simulink model "Passive_balancing"  (R2021a)
settings: Solver=ode23t  StartTime=0.0  StopTime=inf  FixedStep=0.01  MaxStep=0.01  RelTol=1e-3
undefined symbols (not defined in the file): Ion, Lithium
libraries: spsBatteryLib x3, spsIGBTLib x3, spsSeriesRLCBranchLib x3, spspowerguiLib x2
settings Model: PacingRate=79  Creator=AHMED  LastModifiedBy=AHMED

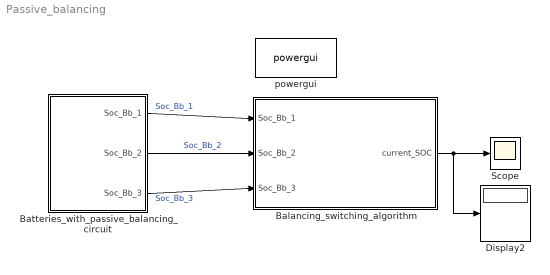
== system Passive_balancing ==
  Balancing_switching_algorithm : Subsystem
  Batteries_with_passive_balancing_circuit : Subsystem  mask{Battery_1_Soc=25, Battery_2_Soc=30, Battery_3_Soc=35}
  Display2 : Display
  Scope : Scope
  powergui : spspowerguiLib/powergui  Priority=1  SimulationMode=Continuous  SampleTime=50e-6  frequency=60  Iterations=50  frequencyindice=0  Pbase=100e6  ErrMax=1e-4  UnitsV=kV  UnitsW=MW  buscounter=0  FunctionMessages=off  echomessages=off  EnableUseOfTLC=off  CurrentSourceSwitches=off  DisableSnubberDevices=off  DisableRonSwitches=off  DisableVfSwitches=off  DisplayEquations=off  AutomaticDiscreteSolvers=off  SolverType=Tustin/Backward Euler (TBE)  Interpol=off  ExternalGateDelay=off  methode=off  Ts=100  x0status=blocks  SPID=on  SwTol=0  HookPort=off  NonlinearTolerance=1e-4  nMaxIteration=100  ContinueOnMaxIteration=off  RestoreLinks=warning  ResistiveCurrentMeasurement=off  Frange=[0:2:500]  Ylog=off  Xlog=on  ShowGrid=off  save=off  variable=ZData  structure=0  ZoomFFT=off  StartTime=0.0  cycles=1  DisplayStyle=1  fundamental=60  FreqAxis=off  MaxFrequency=1000  frequencyindicesteady=1  RmsSteady=1  display=off
  wires:
  Balancing_switching_algorithm/1(current_SOC) -> Display2/1, Scope/1
  Batteries_with_passive_balancing_circuit/1(Soc_Bb_1) -> Balancing_switching_algorithm/1(Soc_Bb_1)  "Soc_Bb_1"
  Batteries_with_passive_balancing_circuit/2(Soc_Bb_2) -> Balancing_switching_algorithm/2(Soc_Bb_2)  "Soc_Bb_2"
  Batteries_with_passive_balancing_circuit/3(Soc_Bb_3) -> Balancing_switching_algorithm/3(Soc_Bb_3)  "Soc_Bb_3"

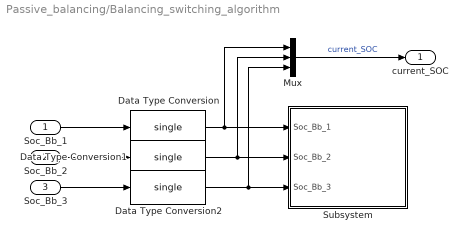
== system Passive_balancing/Balancing_switching_algorithm ==
  Soc_Bb_1 : Inport
  Soc_Bb_2 : Inport  Port=2
  Soc_Bb_3 : Inport  Port=3
  Data Type Conversion : DataTypeConversion  OutDataTypeStr=single
  Data Type Conversion1 : DataTypeConversion  OutDataTypeStr=single
  Data Type Conversion2 : DataTypeConversion  OutDataTypeStr=single
  Mux : Mux  Inputs=3
  Subsystem : Subsystem
  current_SOC : Outport
  wires:
  Data Type Conversion/1 -> Subsystem/1(Soc_Bb_1), Mux/1
  Data Type Conversion1/1 -> Subsystem/2(Soc_Bb_2), Mux/2
  Soc_Bb_3/1 -> Data Type Conversion2/1
  Data Type Conversion2/1 -> Subsystem/3(Soc_Bb_3), Mux/3
  Soc_Bb_2/1 -> Data Type Conversion1/1
  Mux/1 -> current_SOC/1  "current_SOC"
  Soc_Bb_1/1 -> Data Type Conversion/1

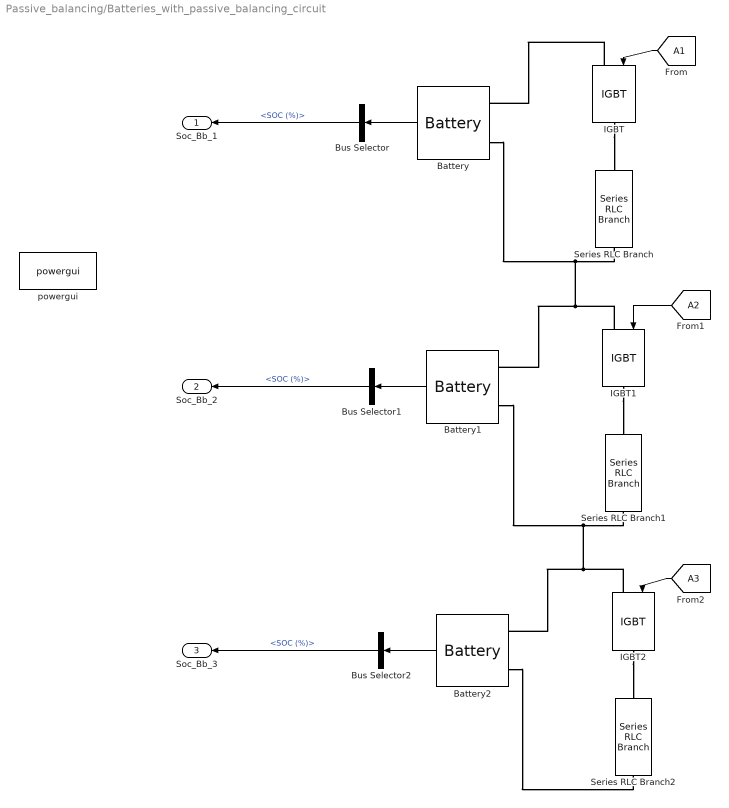
== system Passive_balancing/Batteries_with_passive_balancing_circuit ==
  Battery : spsBatteryLib/Battery  BatType=Lithium-Ion  ShowTempParam=off  ThermalPreset=no  ShowAgeParam=off  NomV=3.7  NomQ=5.4  SOC=Battery_1_Soc  Batt_Tr=30  PresetModel=on  MaxQ=5.4  MinV=2.775  FullV=4.3068  Dis_rate=2.3478  R=0.0068519  Normal_OP=4.8835  expZone="[3.9974      0.2653]"  current=[6.5 13 32.5]  Units=Time  Tci=20  NomT=20  T2=-30  MaxQ2=4.8  FullV2=7.1  Normal_OP2=5.655  expZone2="[6.58           1]"  Rca=0.6  ti=2000  Dp=0  Neq0=0  Tsim=1e6  Ta1=25  Qeol=5.4*0.9  Reol=0.013333*1.2  Char_age=[2.3478, 3]  Dis_age=[2.3478, 10]  N1=1500  N2=10500  N3=1000  N4=1400  Ta2=45  N5=950
  Battery1 : spsBatteryLib/Battery  BatType=Lithium-Ion  ShowTempParam=off  ThermalPreset=no  ShowAgeParam=off  NomV=3.7  NomQ=5.4  SOC=Battery_2_Soc  Batt_Tr=30  PresetModel=on  MaxQ=5.4  MinV=2.775  FullV=4.3068  Dis_rate=2.3478  R=0.0068519  Normal_OP=4.8835  expZone="[3.9974      0.2653]"  current=[6.5 13 32.5]  Units=Time  Tci=20  NomT=20  T2=-30  MaxQ2=4.8  FullV2=7.1  Normal_OP2=5.655  expZone2="[6.58           1]"  Rca=0.6  ti=2000  Dp=0  Neq0=0  Tsim=1e6  Ta1=25  Qeol=5.4*0.9  Reol=0.013333*1.2  Char_age=[2.3478, 3]  Dis_age=[2.3478, 10]  N1=1500  N2=10500  N3=1000  N4=1400  Ta2=45  N5=950
  Battery2 : spsBatteryLib/Battery  BatType=Lithium-Ion  ShowTempParam=off  ThermalPreset=no  ShowAgeParam=off  NomV=3.7  NomQ=5.4  SOC=Battery_3_Soc  Batt_Tr=30  PresetModel=on  MaxQ=5.4  MinV=2.775  FullV=4.3068  Dis_rate=2.3478  R=0.0068519  Normal_OP=4.8835  expZone="[3.9974      0.2653]"  current=[6.5 13 32.5]  Units=Time  Tci=20  NomT=20  T2=-30  MaxQ2=4.8  FullV2=7.1  Normal_OP2=5.655  expZone2="[6.58           1]"  Rca=0.6  ti=2000  Dp=0  Neq0=0  Tsim=1e6  Ta1=25  Qeol=5.4*0.9  Reol=0.013333*1.2  Char_age=[2.3478, 3]  Dis_age=[2.3478, 10]  N1=1500  N2=10500  N3=1000  N4=1400  Ta2=45  N5=950
  Bus Selector : BusSelector  OutputSignals=SOC (%)
  Bus Selector1 : BusSelector  OutputSignals=SOC (%)
  Bus Selector2 : BusSelector  OutputSignals=SOC (%)
  IGBT : spsIGBTLib/IGBT  Ron=0.001  Lon=0  Vf=1  Tf=1e-6  Tt=2e-6  IC=0  Rs=1e5  Cs=inf  Measurements=off
  IGBT1 : spsIGBTLib/IGBT  Ron=0.001  Lon=0  Vf=1  Tf=1e-6  Tt=2e-6  IC=0  Rs=1e5  Cs=inf  Measurements=off
  IGBT2 : spsIGBTLib/IGBT  Ron=0.001  Lon=0  Vf=1  Tf=1e-6  Tt=2e-6  IC=0  Rs=1e5  Cs=inf  Measurements=off
  Series RLC Branch : spsSeriesRLCBranchLib/Series RLC Branch  LConnTagsString=__new0  RConnTagsString=__new0  BranchType=R  Resistance=1  Inductance=1e-3  SetiL0=off  InitialCurrent=0  Capacitance=1e-6  Setx0=off  InitialVoltage=0  Measurements=None
  Series RLC Branch1 : spsSeriesRLCBranchLib/Series RLC Branch  LConnTagsString=__new0  RConnTagsString=__new0  BranchType=R  Resistance=1  Inductance=1e-3  SetiL0=off  InitialCurrent=0  Capacitance=1e-6  Setx0=off  InitialVoltage=0  Measurements=None
  Series RLC Branch2 : spsSeriesRLCBranchLib/Series RLC Branch  LConnTagsString=__new0  RConnTagsString=__new0  BranchType=R  Resistance=1  Inductance=1e-3  SetiL0=off  InitialCurrent=0  Capacitance=1e-6  Setx0=off  InitialVoltage=0  Measurements=None
  powergui : spspowerguiLib/powergui  Priority=1  SimulationMode=Continuous  SampleTime=50e-6  frequency=60  Iterations=50  frequencyindice=0  Pbase=100e6  ErrMax=1e-4  UnitsV=kV  UnitsW=MW  buscounter=0  FunctionMessages=off  echomessages=off  EnableUseOfTLC=off  CurrentSourceSwitches=off  DisableSnubberDevices=off  DisableRonSwitches=off  DisableVfSwitches=off  DisplayEquations=off  AutomaticDiscreteSolvers=off  SolverType=Tustin/Backward Euler (TBE)  Interpol=off  ExternalGateDelay=off  methode=off  Ts=100  x0status=blocks  SPID=on  SwTol=0  HookPort=off  NonlinearTolerance=1e-4  nMaxIteration=100  ContinueOnMaxIteration=off  RestoreLinks=warning  ResistiveCurrentMeasurement=off  Frange=[0:2:500]  Ylog=off  Xlog=on  ShowGrid=off  save=off  variable=ZData  structure=0  ZoomFFT=off  StartTime=0.0  cycles=1  DisplayStyle=1  fundamental=60  FreqAxis=off  MaxFrequency=1000  frequencyindicesteady=1  RmsSteady=1  display=off
  Soc_Bb_1 : Outport
  Soc_Bb_2 : Outport  Port=2
  Soc_Bb_3 : Outport  Port=3
  wires:
  [A1] -> IGBT/1
  Battery/1 -> Bus Selector/1
  [A2] -> IGBT1/1
  Battery2/1 -> Bus Selector2/1
  Bus Selector1/1 -> Soc_Bb_2/1  "<SOC (%)>"
  Battery1/1 -> Bus Selector1/1
  [A3] -> IGBT2/1
  Bus Selector/1 -> Soc_Bb_1/1  "<SOC (%)>"
  Bus Selector2/1 -> Soc_Bb_3/1  "<SOC (%)>"
  connections:
  IGBT1/LConn1 -- Battery1/LConn1 -- Battery/LConn2 -- Series RLC Branch/RConn1
  IGBT2/LConn1 -- Battery2/LConn1 -- Series RLC Branch1/RConn1 -- Battery1/LConn2
  Battery2/LConn2 -- Series RLC Branch2/RConn1
  IGBT/RConn1 -- Series RLC Branch/LConn1
  IGBT/LConn1 -- Battery/LConn1
  IGBT1/RConn1 -- Series RLC Branch1/LConn1
  IGBT2/RConn1 -- Series RLC Branch2/LConn1

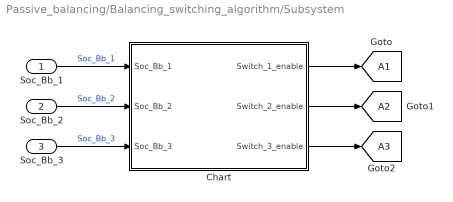
== system Passive_balancing/Balancing_switching_algorithm/Subsystem ==
  Soc_Bb_1 : Inport
  Soc_Bb_2 : Inport  Port=2
  Soc_Bb_3 : Inport  Port=3
  Chart : Stateflow chart  TreatAsAtomicUnit=on
  tag scope: A1=global, A2=global, A3=global
  wires:
  Soc_Bb_1/1 -> Chart/1(Soc_Bb_1)  "Soc_Bb_1"
  Soc_Bb_2/1 -> Chart/2(Soc_Bb_2)  "Soc_Bb_2"
  Soc_Bb_3/1 -> Chart/3(Soc_Bb_3)  "Soc_Bb_3"
  Chart/1(Switch_1_enable) -> [A1]
  Chart/2(Switch_2_enable) -> [A2]
  Chart/3(Switch_3_enable) -> [A3]

== stateflow chart Passive_balancing/Balancing_switching_algorithm/Subsystem/Chart ==
  state First_battery [parallel]
    settings: executionOrder=1
    First_battery -> (junction 19)
    (junction 19) -> (junction 20) [order 1] : [(Soc_Bb_1>Soc_Bb_2)||(Soc_Bb_1>Soc_Bb_3)]
    (junction 19) -> (junction 13) [order 2] : {Switch_1_enable=0;}
    (junction 20) -> (junction 21) : {Switch_1_enable=1;}
    (junction 21) -> (junction 13)
    (junction 13) -> (junction 22)
  state Second_battery [parallel]
    settings: executionOrder=2
    Second_battery -> (junction 34)
    (junction 34) -> (junction 32) [order 1] : [(Soc_Bb_2>Soc_Bb_1)||(Soc_Bb_2>Soc_Bb_3)]
    (junction 34) -> (junction 36) [order 2] : {Switch_2_enable=0;}
    (junction 32) -> (junction 26) : {Switch_2_enable=1;}
    (junction 26) -> (junction 36)
    (junction 36) -> (junction 27)
  state Third_battery [parallel]
    settings: executionOrder=3
    Third_battery -> (junction 3)
    (junction 3) -> (junction 6) [order 1] : [(Soc_Bb_3>Soc_Bb_2)||(Soc_Bb_3>Soc_Bb_1)]
    (junction 3) -> (junction 2) [order 2] : {Switch_3_enable=0;}
    (junction 6) -> (junction 9) : {Switch_3_enable=1;}
    (junction 9) -> (junction 2)
    (junction 2) -> (junction 4)
  data: Soc_Bb_1 input; Soc_Bb_2 input; Soc_Bb_3 input; Switch_1_enable output; Switch_2_enable output double; Switch_3_enable output double
